simulink model "furuta_open_loop"  (R2025a)
settings: Solver=VariableStepAuto  StartTime=0.0  StopTime=50.00  RelTol=1e-3
libraries: cstblocks x1, simulink x1
settings Model: Creator=kales  LastModifiedBy=kales

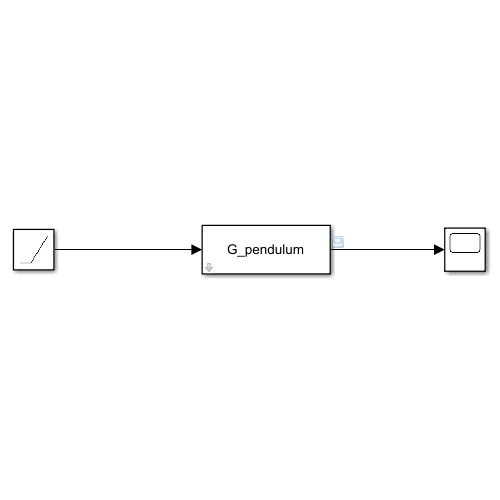
[thumbnail: Simulink's stored preview of the top-level diagram]
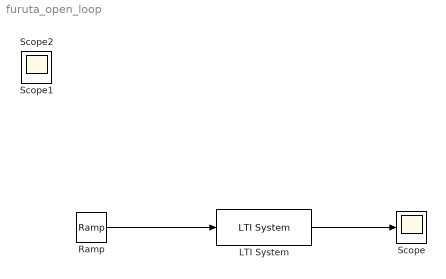
== system furuta_open_loop ==
  LTI System : cstblocks/LTI System  sys=G_pendulum  IC=[]  PadeOrder=0
  Ramp : simulink/Sources/Ramp  slope=1  start=0  InitialOutput=0
  Scope : Scope
      settings: ActiveDisplayYMinimum=-1.1083000726760995E+161  ActiveDisplayYMaximum=7.4311735699576342E+161
  Scope1 : Scope
      settings: ActiveDisplayYMinimum=-1.8009797374561778E+42  ActiveDisplayYMaximum=2.5290301752241046E+42
  Scope2 : Scope
      settings: ActiveDisplayYMinimum=-0.42456381260640885  ActiveDisplayYMaximum=1.7133603850389849  DataLoggingVariableName=ScopeData2
  wires:
  Ramp/1 -> LTI System/1
  LTI System/1 -> Scope/1
